simulink model "grandland_sim_2"  (R2023b)
settings: Solver=VariableStepAuto  StartTime=0.0  StopTime=2  RelTol=1e-3
StartFcn:
  | clear grandland_controller;
values from neighbouring files (symbols this model uses):
  Ts = 0.01    [grandland.m]    (also in grandland_3.m = 0.02; test.m)
libraries: cstblocks x9
settings Model: Creator=antor  LastModifiedBy=antor

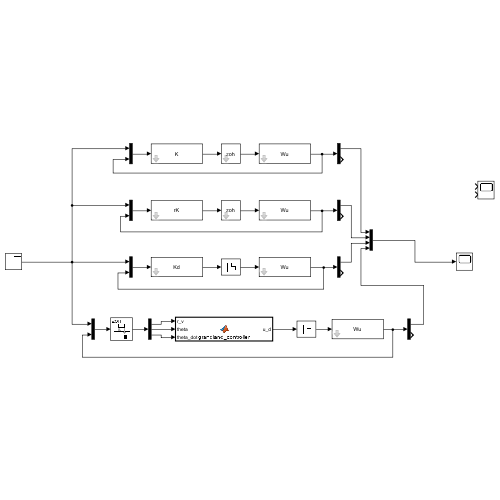
[thumbnail: Simulink's stored preview of the top-level diagram]
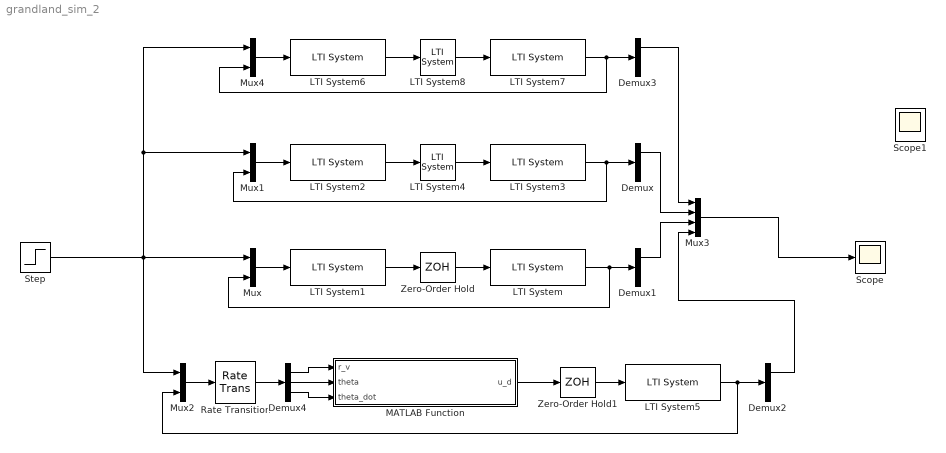
== system grandland_sim_2 ==
  Demux{,1..3} (4 alike) : Demux  Outputs=2
  Demux4 : Demux  Outputs=3
  LTI System{,3,5,7} (4 alike) : cstblocks/LTI System  sys=Wu  IC=[]  PadeOrder=0
  LTI System1 : cstblocks/LTI System  sys=Kd  IC=[]  PadeOrder=0
  LTI System2 : cstblocks/LTI System  sys=rK  IC=[]  PadeOrder=0
  LTI System4 : cstblocks/LTI System  sys=zoh  IC=[]  PadeOrder=0
  LTI System6 : cstblocks/LTI System  sys=K  IC=[]  PadeOrder=0
  LTI System8 : cstblocks/LTI System  sys=zoh  IC=[]  PadeOrder=0
  MATLAB Function : MATLAB Function  TreatAsAtomicUnit=on
  Mux{,1..2,4} (4 alike) : Mux  Inputs=2
  Mux3 : Mux
  Rate Transition : RateTransition  OutPortSampleTime=Ts
  Scope : Scope
  Scope1 : Scope  NumInputPorts=2
  Step : Step  Time=0  After=0.1  SampleTime=0
  Zero-Order Hold : ZeroOrderHold  SampleTime=Ts
  Zero-Order Hold1 : ZeroOrderHold  SampleTime=Ts
  wires:
  Zero-Order Hold/1 -> LTI System/1
  LTI System1/1 -> Zero-Order Hold/1
  LTI System/1 -> Demux1/1, Mux/2
  Mux/1 -> LTI System1/1
  LTI System3/1 -> Demux/1, Mux1/2
  Mux1/1 -> LTI System2/1
  LTI System2/1 -> LTI System4/1
  LTI System4/1 -> LTI System3/1
  Demux/1 -> Mux3/2
  Demux1/1 -> Mux3/3
  Zero-Order Hold1/1 -> LTI System5/1
  Mux2/1 -> Rate Transition/1
  LTI System5/1 -> Mux2/2, Demux2/1
  Demux2/1 -> Mux3/4
  Demux3/1 -> Mux3/1
  Mux4/1 -> LTI System6/1
  LTI System7/1 -> Demux3/1, Mux4/2
  Step/1 -> Mux4/1, Mux1/1, Mux2/1, Mux/1
  LTI System8/1 -> LTI System7/1
  LTI System6/1 -> LTI System8/1
  Mux3/1 -> Scope/1
  Rate Transition/1 -> Demux4/1
  Demux4/1 -> MATLAB Function/1(r_v)
  Demux4/2 -> MATLAB Function/2(theta)
  Demux4/3 -> MATLAB Function/3(theta_dot)
  MATLAB Function/1(u_d) -> Zero-Order Hold1/1

== matlab function grandland_sim_2/MATLAB Function ==
  settings: updateMethod=DISCRETE
  data: Kd_coeff parameter; r_v input; theta input; theta_dot input; u_d output
function u_d = grandland_controller(Kd_coeff, r_v, theta, theta_dot)

persistent state;
if isempty(state)
    state = zeros(4, 3);
end

state(:, 2:3) = state(:, 1:2);
state(1:3, 1) = [r_v; theta; theta_dot];

u_d = 0;
for i = 1:3
    num = Kd_coeff(i, 1:3);
    u_d = u_d+(num(1)*state(i, 1)+num(2)*state(i, 2)+num(3)*state(i, 3));
end
den = Kd_coeff(i+1, 1:3);
u_d = u_d-den(2)*state(4, 2)-den(3)*state(4, 3);

state(4, 1) = u_d;

end
